simulink subsystem "acq_PNR"  (R2019b)
settings: Solver=VariableStepAuto  StartTime=0.0  StopTime=10.0  RelTol=1e-3
undefined symbols (not defined in the file): __PRM__SERIALIZED__DATA__, freq_vector, SubsystemReferenceBlock
libraries: simulink x1, dspstat3 x1
settings Model: Creator=nishantmittal  LastModifiedBy=nishantmittal

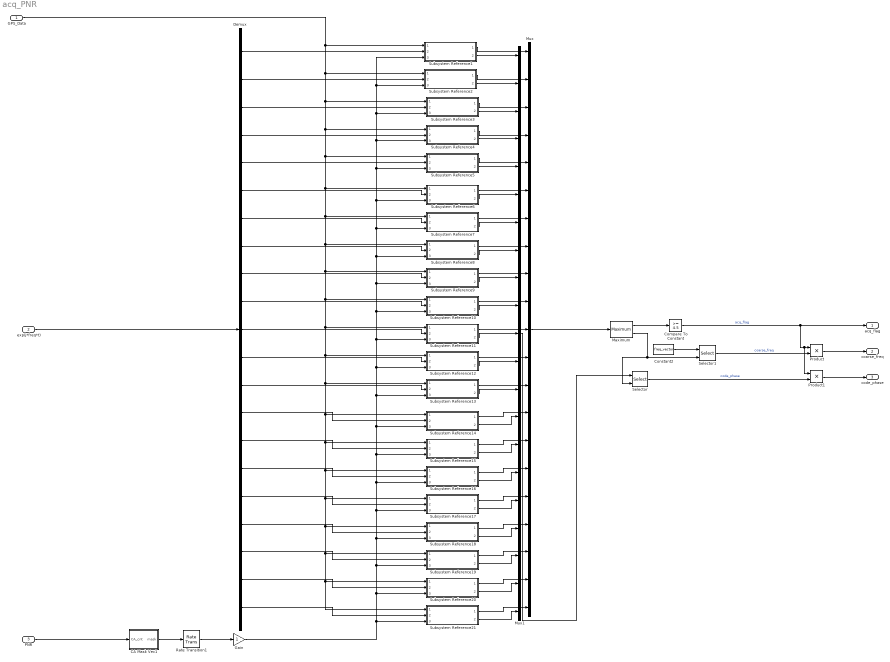
== system acq_PNR ==
  GPS_Data : Inport
  exp(j*freq*t) : Inport  Port=2
  PNR : Inport  Port=3
  CA Mask Vec1 : MATLAB Function  TreatAsAtomicUnit=on
  Compare To Constant : simulink/Logic and Bit Operations/Compare To Constant  relop=>=  const=4.5  OutDataTypeStr=boolean
  Constant2 : Constant  Value=freq_vector  OutDataTypeStr=single
  Demux : Demux  Outputs=21
  Gain : Gain  OutDataTypeStr=uint8
  Maximum : dspstat3/Maximum  operation=maximum  fcn=Value and Index  indexBase=One  operateOver=Each column  Dimension=1  InputProcessing=Columns as channels (frame based)  reset=None  roiEnable=off  roiType=Rectangles  roiPortion=Entire ROI  roiOutput=Individual statistics for each ROI  roiFlag=off  roundingMode=Floor  overflowMode=off  accumDataTypeStr=Inherit: Same as product output  accumLastDataTypeStr=Inherit: Same as product output
  Mux : Mux  Inputs=21
  Mux1 : Mux  Inputs=21
  Product : Product
  Product1 : Product
  Rate Transition1 : RateTransition  Deterministic=off  OutPortSampleTime=1/(1.023e6)
  Selector : Selector  InputPortWidth=21  IndexOptions=Index vector (port)  Indices=[1 3]  OutputSizes=1
  Selector1 : Selector  InputPortWidth=21  IndexOptions=Index vector (port)  Indices=[1 3]  OutputSizes=1
  Subsystem Reference{1..21} (21 alike) : Subsystem  BlockKeywords=__PRM__SERIALIZED__DATA__:SubsystemReferenceBlock  ReferencedSubsystem=acq_block
  acq_flag : Outport
  coarse_freq : Outport  Port=2
  code_phase : Outport  Port=3
  wires:
  Mux1/1 -> Selector/1
  Subsystem Reference1/2 -> Mux1/1
  Compare To Constant/1 -> acq_flag/1, Product/1, Product1/1  "acq_flag"
  Demux/14 -> Subsystem Reference14/2
  Demux/10 -> Subsystem Reference10/2
  Maximum/2 -> Selector1/2, Selector/2
  Subsystem Reference11/2 -> Mux1/11
  Subsystem Reference16/2 -> Mux1/16
  Subsystem Reference18/2 -> Mux1/18
  Demux/6 -> Subsystem Reference6/2
  Rate Transition1/1 -> Gain/1
  GPS_Data/1 -> Subsystem Reference2/1, Subsystem Reference3/1, Subsystem Reference4/1, Subsystem Reference5/1, Subsystem Reference6/1, Subsystem Reference7/1, Subsystem Reference8/1, Subsystem Reference9/1, Subsystem Reference10/1, Subsystem Reference11/1, Subsystem Reference12/1, Subsystem Reference13/1, Subsystem Reference14/1, Subsystem Reference15/1, Subsystem Reference16/1, Subsystem Reference17/1, Subsystem Reference18/1, Subsystem Reference19/1, Subsystem Reference21/1, Subsystem Reference20/1, Subsystem Reference1/1
  Subsystem Reference3/1 -> Mux/3
  Demux/12 -> Subsystem Reference12/2
  Constant2/1 -> Selector1/1
  Demux/16 -> Subsystem Reference16/2
  Subsystem Reference18/1 -> Mux/18
  Subsystem Reference2/1 -> Mux/2
  Subsystem Reference19/1 -> Mux/19
  Subsystem Reference7/2 -> Mux1/7
  Subsystem Reference11/1 -> Mux/11
  Subsystem Reference15/2 -> Mux1/15
  Subsystem Reference14/2 -> Mux1/14
  PNR/1 -> CA Mask Vec1/1(CA_cnt)
  Subsystem Reference1/1 -> Mux/1
  exp(j*freq*t)/1 -> Demux/1
  Subsystem Reference12/1 -> Mux/12
  Subsystem Reference20/1 -> Mux/20
  Subsystem Reference21/1 -> Mux/21
  Subsystem Reference2/2 -> Mux1/2
  Demux/20 -> Subsystem Reference20/2
  Demux/19 -> Subsystem Reference19/2
  Demux/2 -> Subsystem Reference2/2
  Demux/7 -> Subsystem Reference7/2
  Subsystem Reference6/1 -> Mux/6
  Gain/1 -> Subsystem Reference21/3, Subsystem Reference20/3, Subsystem Reference19/3, Subsystem Reference18/3, Subsystem Reference17/3, Subsystem Reference16/3, Subsystem Reference15/3, Subsystem Reference14/3, Subsystem Reference13/3, Subsystem Reference12/3, Subsystem Reference11/3, Subsystem Reference10/3, Subsystem Reference9/3, Subsystem Reference8/3, Subsystem Reference7/3, Subsystem Reference6/3, Subsystem Reference5/3, Subsystem Reference4/3, Subsystem Reference3/3, Subsystem Reference2/3, Subsystem Reference1/3
  Subsystem Reference8/2 -> Mux1/8
  Subsystem Reference10/1 -> Mux/10
  Subsystem Reference10/2 -> Mux1/10
  Subsystem Reference4/2 -> Mux1/4
  Subsystem Reference19/2 -> Mux1/19
  Selector/1 -> Product1/2  "code_phase"
  Mux/1 -> Maximum/1
  Subsystem Reference13/2 -> Mux1/13
  Subsystem Reference17/2 -> Mux1/17
  CA Mask Vec1/1(mask) -> Rate Transition1/1
  Subsystem Reference21/2 -> Mux1/21
  Demux/18 -> Subsystem Reference18/2
  Demux/21 -> Subsystem Reference21/2
  Subsystem Reference3/2 -> Mux1/3
  Demux/4 -> Subsystem Reference4/2
  Subsystem Reference5/1 -> Mux/5
  Subsystem Reference7/1 -> Mux/7
  Subsystem Reference9/2 -> Mux1/9
  Subsystem Reference9/1 -> Mux/9
  Demux/9 -> Subsystem Reference9/2
  Subsystem Reference17/1 -> Mux/17
  Demux/11 -> Subsystem Reference11/2
  Demux/1 -> Subsystem Reference1/2
  Subsystem Reference13/1 -> Mux/13
  Subsystem Reference5/2 -> Mux1/5
  Subsystem Reference20/2 -> Mux1/20
  Demux/15 -> Subsystem Reference15/2
  Subsystem Reference14/1 -> Mux/14
  Demux/17 -> Subsystem Reference17/2
  Subsystem Reference6/2 -> Mux1/6
  Demux/13 -> Subsystem Reference13/2
  Demux/5 -> Subsystem Reference5/2
  Selector1/1 -> Product/2  "coarse_freq"
  Demux/8 -> Subsystem Reference8/2
  Subsystem Reference8/1 -> Mux/8
  Subsystem Reference16/1 -> Mux/16
  Demux/3 -> Subsystem Reference3/2
  Maximum/1 -> Compare To Constant/1
  Subsystem Reference15/1 -> Mux/15
  Subsystem Reference4/1 -> Mux/4
  Subsystem Reference12/2 -> Mux1/12
  Product1/1 -> code_phase/1
  Product/1 -> coarse_freq/1

== matlab function acq_PNR/CA Mask Vec1 ==
  data: CA_cnt input; mask output
function mask = fcn(CA_cnt)

phase = [2 6; 3 7; 4 8; 5 9; 1 9; 2 10; 1 8; 2 9; 3 10; 2 3; 3 4; 5 6; 6 7; 7 8; 8 9; 9 10; 1 4; 2 5; 3 6; 4 7; 5 8; 6 9; 1 3; 4 6; 5 7; 6 8; 7 9; 8 10; 1 6; 2 7; 3 8; 4 9];
mask_points = phase(CA_cnt, :);
mask = zeros(1,10);
mask(mask_points) = 1;
